simulink model "Project5_Quiz"  (R2014a)
settings: Solver=ode45  StartTime=0.0  StopTime=3600  RelTol=1e-3
undefined symbols (not defined in the file): i, OCV, Q, R_Charging, R_Discharging, SOC
settings Model: Creator=DZR3QN  LastModifiedBy=DZR3QN

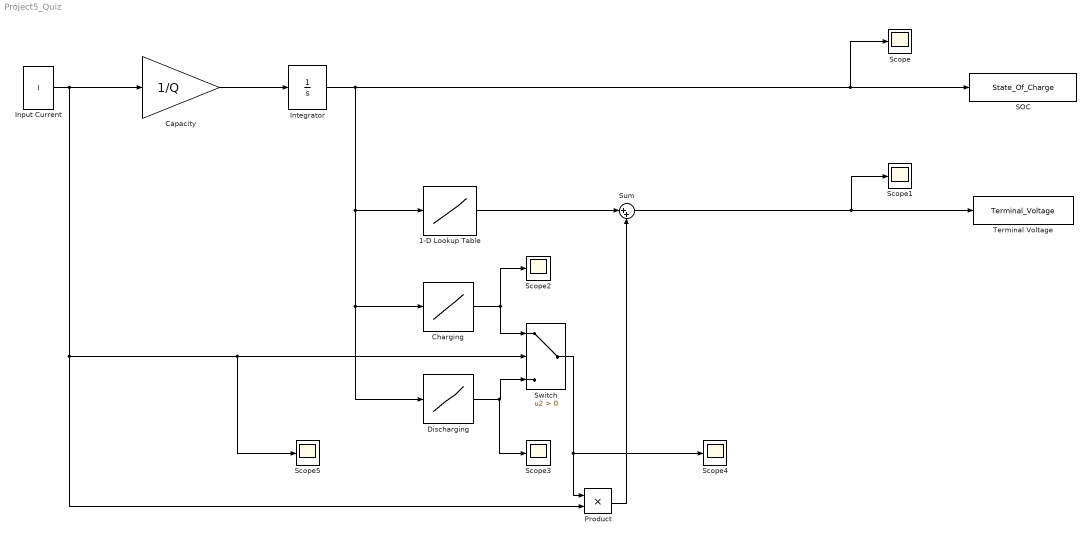
== system Project5_Quiz ==
  1-D Lookup Table : Lookup_n-D  NumberOfTableDimensions=1  BreakpointsForDimension1=SOC  Table=OCV  InternalRulePriority=Speed  RndMeth=Simplest  InputSameDT=on
  Capacity : Gain  Gain=1/Q
  Charging : Lookup_n-D  NumberOfTableDimensions=1  BreakpointsForDimension1=SOC  Table=R_Charging  InternalRulePriority=Speed  RndMeth=Simplest  InputSameDT=on
  Discharging : Lookup_n-D  NumberOfTableDimensions=1  BreakpointsForDimension1=SOC  Table=R_Discharging  InternalRulePriority=Speed  RndMeth=Simplest  InputSameDT=on
  Input Current : Constant  Value=i
  Integrator : Integrator
  Product : Product  RndMeth=Zero
  SOC : ToWorkspace  VariableName=State_Of_Charge  SaveFormat=Structure  SampleTime=-1
  Scope{,1..5} (6 alike) : Scope
      Scope2 settings: SaveName=ScopeData2
      Scope3 settings: SaveName=ScopeData3
      Scope4 settings: SaveName=ScopeData4
      Scope5 settings: SaveName=ScopeData5
  Sum : Sum  Inputs=|++
  Switch : Switch  Criteria=u2 > Threshold
  Terminal Voltage : ToWorkspace  VariableName=Terminal_Voltage  SaveFormat=Structure  SampleTime=-1
  wires:
  Capacity/1 -> Integrator/1
  Input Current/1 -> Scope5/1, Switch/2, Product/2, Capacity/1
  Integrator/1 -> Discharging/1, Charging/1, 1-D Lookup Table/1, Scope/1, SOC/1
  Product/1 -> Sum/2
  1-D Lookup Table/1 -> Sum/1
  Sum/1 -> Scope1/1, Terminal Voltage/1
  Charging/1 -> Scope2/1, Switch/1
  Discharging/1 -> Scope3/1, Switch/3
  Switch/1 -> Scope4/1, Product/1
